simulink model "Test1_3"  (R2021a)
(part 2 of 2)

  Line 71/RConn3 -- Load 8041/LConn3
  Line 38/RConn1 -- Load 13/LConn1
  Line 38/RConn2 -- Load 13/LConn2
  Line 38/RConn3 -- Load 13/LConn3
  Line 15/RConn1 -- Load 6/LConn1
  Line 15/RConn2 -- Load 6/LConn2
  Line 15/RConn3 -- Load 6/LConn3
  Line 49/LConn1 -- Line 48/LConn1 -- Line 47/RConn1
  Line 49/LConn2 -- Line 48/LConn2 -- Line 47/RConn2
  Line 49/LConn3 -- Line 48/LConn3 -- Line 47/RConn3
  Line 1/RConn1 -- R3/LConn1
  Line 1/RConn2 -- R3/LConn2
  Line 1/RConn3 -- R3/LConn3
  Load 11/LConn1 -- Line 32/RConn1
  Load 11/LConn2 -- Line 32/RConn2
  Load 11/LConn3 -- Line 32/RConn3
  Line im1/LConn1 -- R3/RConn1
  Line im1/LConn2 -- R3/RConn2
  Line im1/LConn3 -- R3/RConn3
  Line 72/LConn1 -- Line 73/RConn1
  Line 72/LConn2 -- Line 73/RConn2
  Line 72/LConn3 -- Line 73/RConn3
  Line 24/RConn1 -- Line 25/LConn1
  Line 24/RConn2 -- Line 25/LConn2
  Line 24/RConn3 -- Line 25/LConn3
  Line 52/LConn1 -- Line 51/LConn1 -- Line 53/RConn1
  Line 52/LConn2 -- Line 51/LConn2 -- Line 53/RConn2
  Line 52/LConn3 -- Line 51/LConn3 -- Line 53/RConn3
  Line 69/RConn1 -- Load 8287/LConn1
  Line 69/RConn2 -- Load 8287/LConn2
  Line 69/RConn3 -- Load 8287/LConn3
  Line 60/LConn1 -- Line 59/LConn1 -- Line im1/RConn1
  Line 60/LConn2 -- Line 59/LConn2 -- Line im1/RConn2
  Line 60/LConn3 -- Line 59/LConn3 -- Line im1/RConn3
  Line 17/LConn1 -- Line 18/RConn1
  Line 17/LConn2 -- Line 18/RConn2
  Line 17/LConn3 -- Line 18/RConn3
  Load 8733/LConn1 -- Line 63/RConn1
  Load 8733/LConn2 -- Line 63/RConn2
  Load 8733/LConn3 -- Line 63/RConn3
  Line 10/RConn1 -- Load 1/LConn1
  Line 10/RConn2 -- Load 1/LConn2
  Line 10/RConn3 -- Load 1/LConn3
  Line 18/LConn1 -- Line im3/RConn1
  Line 18/LConn2 -- Line im3/RConn2
  Line 18/LConn3 -- Line im3/RConn3
  Line 71/LConn1 -- Line 70/LConn1 -- Line 72/RConn1
  Line 71/LConn2 -- Line 70/LConn2 -- Line 72/RConn2
  Line 71/LConn3 -- Line 70/LConn3 -- Line 72/RConn3
  Line 27/RConn1 -- R4/LConn1
  Line 27/RConn2 -- R4/LConn2
  Line 27/RConn3 -- R4/LConn3
